simulink model "test_setProblem_ineqConst"  (R2018a)
settings: Solver=FixedStepAuto  StartTime=0.0  StopTime=inf  FixedStep=0.01  RelTol=1e-3
libraries: robotlib x4
settings Model: Creator=bascetta  LastModifiedBy=bascetta
settings OptimizationCC: PassReuseOutputArgsAs=Individual arguments  MaxStackSize=64
settings DebuggingCC: ParameterTunabilityLossMsg=error
settings HardwareCC: ProdBitPerPointer=32  ProdBitPerSizeT=32  ProdBitPerPtrDiffT=32  ProdLargestAtomicFloat=None  ProdIntDivRoundTo=Undefined  ProdEndianess=Unspecified  ProdWordSize=32  ProdHWDeviceType=Generic->Unspecified (assume 32-bit Generic)
settings SFSimCC: SimUserIncludeDirs=./  SimUserLibraries=libCPLEXsolver_cwrapper.so  MATLABDynamicMemAlloc=off
settings RTWCC: SystemTargetFile=ert.tlc  HardwareBoard=Robot Operating System (ROS)  TLCOptions="-aInlineSetEventsForThisBaseRateFcn=TLC_FALSE -aSuppressMultiTaskScheduler=TLC_FALSE  -aRateBasedStepFcn=0"  TemplateMakefile=ert_default_tmf  GenerateReport=on  RTWUseSimCustomCode=on  CustomInclude=./  CustomLibrary=libCPLEXsolver_cwrapper.so  Toolchain=Catkin  IncludeHyperlinkInReport=on  LaunchReport=on  TargetLang=C++  GenerateTraceInfo=on  GenerateTraceReport=on  GenerateTraceReportSl=on  GenerateTraceReportSf=on  GenerateTraceReportEml=on
settings CodeAppCC: ForceParamTrailComments=on  IgnoreCustomStorageClasses=off  OperatorAnnotations=on  SimulinkDataObjDesc=on  SFDataObjDesc=on  MATLABFcnDesc=on  InsertBlockDesc=on  StateflowObjectComments=on  MATLABSourceComments=on
settings ERTTargetCC: SupportContinuousTime=on
settings ConfigComp: CovScope=ReferencedModels  CovIncludeTopModel=off

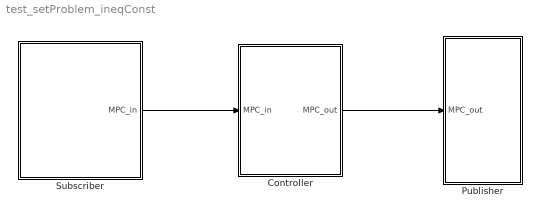
== system test_setProblem_ineqConst ==
  Controller : Subsystem
  Publisher : Subsystem
  "Subscriber " : Subsystem
  wires:
  Controller/1(MPC_out) -> Publisher/1(MPC_out)
  "Subscriber "/1(MPC_in) -> Controller/1(MPC_in)

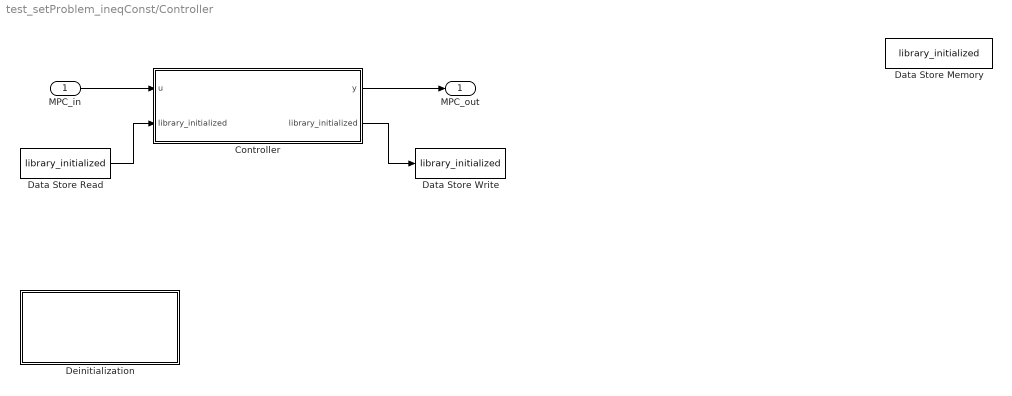
== system test_setProblem_ineqConst/Controller ==
  MPC_in : Inport
  Controller : MATLAB Function  TreatAsAtomicUnit=on
  Data Store Memory : DataStoreMemory  DataStoreName=library_initialized  ReadBeforeWriteMsg=warning  WriteAfterWriteMsg=warning  WriteAfterReadMsg=warning  ShowAdditionalParam=off  OutDataTypeStr=int16
  Data Store Read : DataStoreRead  DataStoreName=library_initialized
  Data Store Write : DataStoreWrite  DataStoreName=library_initialized
  Deinitialization : Subsystem
  MPC_out : Outport
  wires:
  MPC_in/1 -> Controller/1(u)
  Controller/1(y) -> MPC_out/1
  Controller/2(library_initialized) -> Data Store Write/1
  Data Store Read/1 -> Controller/2("library_initialized ")

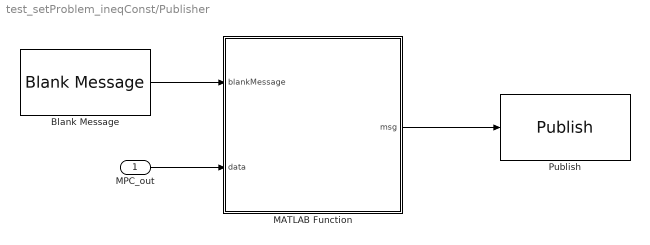
== system test_setProblem_ineqConst/Publisher ==
  MPC_out : Inport
  Blank Message : robotlib/Blank Message  SourceLibraryInfo=This block requires Robotics System Toolbox  messageType=std_msgs/Float64MultiArray  SampleTime=inf
      settings: SourceProductBaseCode=RO
  MATLAB Function : MATLAB Function  TreatAsAtomicUnit=on
  Publish : robotlib/Publish  SourceLibraryInfo=This block requires Robotics System Toolbox  topicSource=Specify your own  topic=/MPC_out  messageType=std_msgs/Float64MultiArray  messageQueueLength=1
      settings: SourceProductBaseCode=RO
  wires:
  Blank Message/1 -> MATLAB Function/1(blankMessage)
  MPC_out/1 -> MATLAB Function/2(data)
  MATLAB Function/1(msg) -> Publish/1

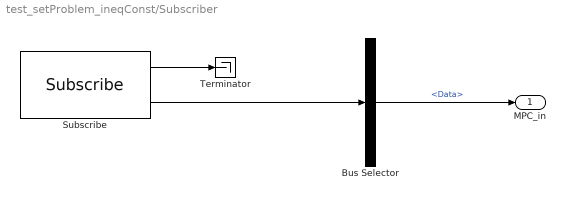
== system test_setProblem_ineqConst/Subscriber  ==
  Bus Selector : BusSelector  OutputSignals=Data
  Subscribe : robotlib/Subscribe  SourceLibraryInfo=This block requires Robotics System Toolbox  topicSource=Specify your own  topic=/MPC_in  messageType=std_msgs/Float64  sampleTime=-1  messageQueueLength=1
      settings: SourceProductBaseCode=RO
  Terminator : Terminator
  MPC_in : Outport
  wires:
  Subscribe/2 -> Bus Selector/1
  Bus Selector/1 -> MPC_in/1  "<Data>"
  Subscribe/1 -> Terminator/1

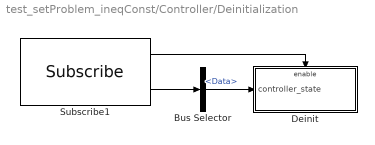
== system test_setProblem_ineqConst/Controller/Deinitialization ==
  Bus Selector : BusSelector  OutputSignals=Data
  Deinit : Subsystem  TreatAsAtomicUnit=on
  Subscribe1 : robotlib/Subscribe  SourceLibraryInfo=This block requires Robotics System Toolbox  topicSource=Specify your own  topic=/controller_state  messageType=std_msgs/Int16  sampleTime=-1  messageQueueLength=1
      settings: SourceProductBaseCode=RO
  wires:
  Subscribe1/1 -> Deinit/Enable
  Subscribe1/2 -> Bus Selector/1
  Bus Selector/1 -> Deinit/1(controller_state)  "<Data>"

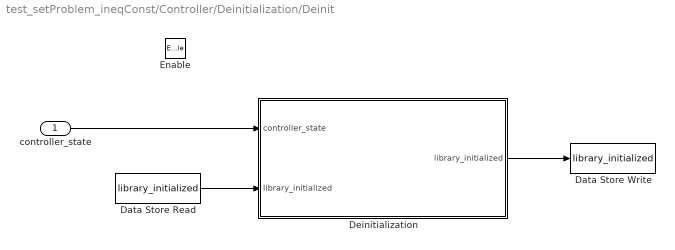
== system test_setProblem_ineqConst/Controller/Deinitialization/Deinit ==
  controller_state : Inport
  Enable : EnablePort
  Data Store Read : DataStoreRead  DataStoreName=library_initialized
  Data Store Write : DataStoreWrite  DataStoreName=library_initialized
  Deinitialization : MATLAB Function  TreatAsAtomicUnit=on
  wires:
  controller_state/1 -> Deinitialization/1(controller_state)
  Data Store Read/1 -> Deinitialization/2("library_initialized ")
  Deinitialization/1(library_initialized) -> Data Store Write/1

== matlab function test_setProblem_ineqConst/Publisher/MATLAB Function ==
  data: blankMessage input; msg output Bus: SL_Bus_test_setProblem_ineqConst_std_msgs_Float64MultiArray; data input
function msg = map_multiArrayMsg(blankMessage,data)

% Assign the output message to be the same with input blank message
msg = blankMessage;

% Modify the nested message
for i=1:length(data)
    msg.Data(i) = data(i);
end

msg.Data_SL_Info.CurrentLength = uint32(length(data));

== matlab function test_setProblem_ineqConst/Controller/Controller ==
  data: u input; y output; library_initialized input; library_initialized output
function [y,library_initialized] = MPC_execute(u,library_initialized)
%#codegen

% Solver library include file
coder.cinclude('CPLEXsolver_cwrapper.h')

%% Initialization
% MPC parameters
numVariable = 3;
numIneqConstraint = 2;
numEqConstraint = 0;
numQIneqConstraint = 0;

% Solver initialization
if (library_initialized == 0)
    coder.ceval('init_CPLEXsolver_cwrapper', int32(numVariable), ...
        int32(numIneqConstraint), int32(numEqConstraint), int32(numQIneqConstraint));

    library_initialized = int16(1);
end

%% Periodic cycle
y = zeros(1,numVariable);

if (library_initialized == 1)
    % Init problem
    coder.ceval('initProblem');

    H = [ 3.0*u,   0.0,   -1.0;
            0.0, 2.0*u,    0.0;
           -1.0,   0.0,  1.0*u ];
    f = [ -2.0, 3.0, 1.0 ];
    A = [ 2.0, 0.0,  1.0;
          0.0, 1.0, -1.0 ];
    b = [ 1.0, -1.0 ]';
    coder.ceval('setProblem_ineqConst', coder.ref(H), coder.ref(f), ...
        coder.ref(A), coder.ref(b));

    % Solve problem
    coder.ceval('solveProblem', coder.wref(y));
end

== matlab function test_setProblem_ineqConst/Controller/Deinitialization/Deinit/Deinitialization ==
  data: controller_state input; library_initialized output; library_initialized input
function library_initialized  = MPC_deinit(controller_state,library_initialized)
%#codegen

if (controller_state <= 0)
    % Solver deinitialization
    if (library_initialized == 1)
        coder.ceval('deinit_CPLEXsolver_cwrapper');
        
        library_initialized = int16(-1);
    end
end

end
